simulink model "Traffic_light_model"  (R2020b)
settings: Solver=VariableStepAuto  StartTime=0.0  StopTime=inf  RelTol=1e-3
settings Model: EnablePacing=on  Creator=ankit  LastModifiedBy=ankit

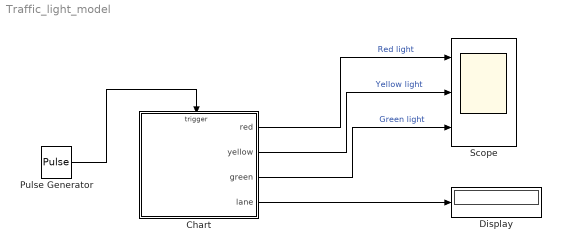
== system Traffic_light_model ==
  Chart : Stateflow chart  TreatAsAtomicUnit=on
  Display : Display
  Pulse Generator : DiscretePulseGenerator  PulseType=Time based  Period=0.001  PulseWidth=25
  Scope : Scope  NumInputPorts=3
  wires:
  Pulse Generator/1 -> Chart/Trigger
  Chart/1(red) -> Scope/1  "Red light"
  Chart/2(yellow) -> Scope/2  "Yellow light"
  Chart/3(green) -> Scope/3  "Green light"
  Chart/4(lane) -> Display/1

== stateflow chart Traffic_light_model/Chart ==
  settings: executeAtInitialization=1
  state Lane2
    en: ctrl = 1;
    lane = 2;
    state redLight
      en: red = 1;
      yellow = 0;
      green = 0;
    state greenLight
      en: red = 0;
      yellow = 0;
      green = 1;
    state yellowLight
      en: red = 0;
      yellow = 1;
      green = 0;
    (default) -> Lane2.redLight
    Lane2.yellowLight -> Lane2.redLight : after(1, sec)/{ctrl = 0}
    Lane2.redLight -> Lane2.greenLight : after(6, sec)[ctrl == 1]
    Lane2.greenLight -> Lane2.yellowLight : after(3, sec)
  state Lane1
    en: ctrl = 1;
    lane = 1;
    state redLight
      en: red = 1;
      yellow = 0;
      green = 0;
    state greenLight
      en: red = 0;
      yellow = 0;
      green = 1;
    state yellowLight
      en: red = 0;
      yellow = 1;
      green = 0;
    (default) -> Lane1.redLight
    Lane1.yellowLight -> Lane1.redLight : after(1, sec)/{ctrl = 0}
    Lane1.redLight -> Lane1.greenLight : after(6, sec)[ctrl == 1]
    Lane1.greenLight -> Lane1.yellowLight : after(3, sec)
  state Lane3
    en: ctrl = 1;
    lane = 3;
    state redLight
      en: red = 1;
      yellow = 0;
      green = 0;
    state greenLight
      en: red = 0;
      yellow = 0;
      green =  1;
    state yellowLight
      en: red = 0;
      yellow = 1;
      green = 0;
    (default) -> Lane3.redLight
    Lane3.yellowLight -> Lane3.redLight : after(1, sec)/{ctrl = 0}
    Lane3.redLight -> Lane3.greenLight : after(6, sec)[ctrl == 1]
    Lane3.greenLight -> Lane3.yellowLight : after(3, sec)
  state Lane4
    en: ctrl = 1;
    lane = 4;
    state redLight
      en: red = 1;
      yellow = 0;
      green = 0;
    state greenLight
      en: red = 0;
      yellow = 0;
      green = 1;
    state yellowLight
      en: red = 0;
      yellow = 1;
      green = 0;
    (default) -> Lane4.redLight
    Lane4.yellowLight -> Lane4.redLight : after(1, sec)/{ctrl = 0}
    Lane4.redLight -> Lane4.greenLight : after(6, sec)[ctrl == 1]
    Lane4.greenLight -> Lane4.yellowLight : after(3, sec)
  Lane2 -> Lane3 : [ctrl == 0]
  Lane1 -> Lane2 : [ctrl == 0]
  (default) -> Lane1
  Lane4 -> Lane1 : [ctrl == 0]
  Lane3 -> Lane4 : [ctrl == 0]
  data: red output; yellow output; green output; ctrl local; lane output
  events: clock input RISING_EDGE_EVENT
